simulink library "CTRL_TRGT_YRUPPB"  (R2023b)
settings: Solver=VariableStepAuto  StartTime=0.0  StopTime=10.0  RelTol=1e-3
undefined symbols (not defined in the file or in its folder): c_GravConst_mps2, CTRL_TRGT_YRUPPB_p_Fct1_na
libraries: VUT_lib x1
settings Model: Creator=blatak  LastModifiedBy=blatak

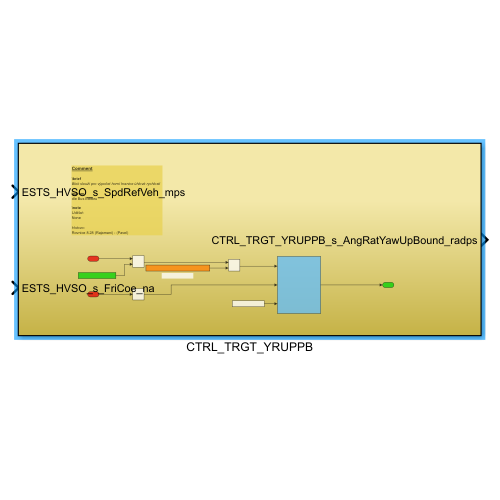
[thumbnail: Simulink's stored preview of the top-level diagram]
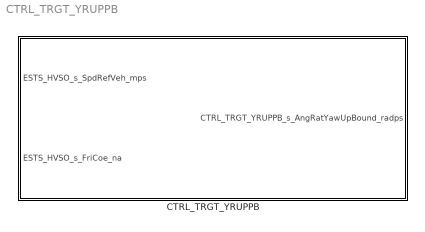
== system CTRL_TRGT_YRUPPB ==
  CTRL_TRGT_YRUPPB : Subsystem

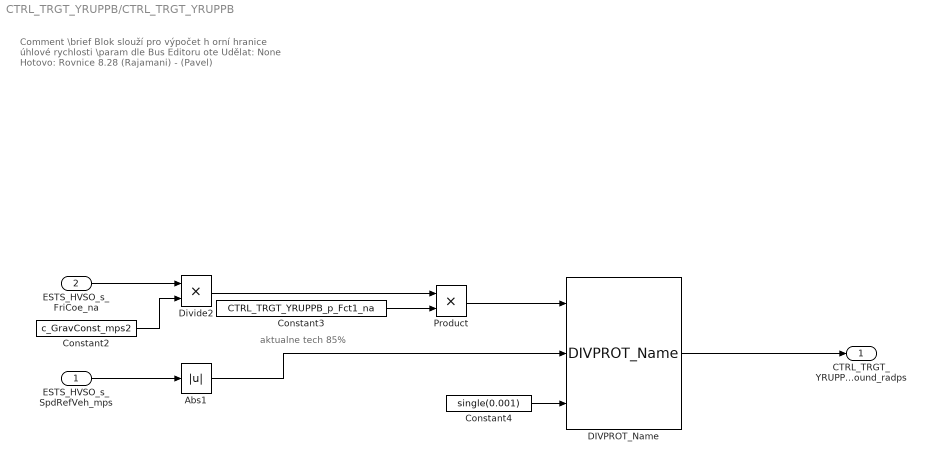
== system CTRL_TRGT_YRUPPB/CTRL_TRGT_YRUPPB ==
  note: aktualne tech 85%
  note: Comment
      |
      | \brief
      | Blok slouží pro výpočet h orní hranice úhlové rychlosti
      |
      | \param
      | dle Bus Editoru
      |
      | \note
      | Udělat:
      | None
      |
      | Hotovo:
      | Rovnice 8.28 (Rajamani) - (Pavel)
  ESTS_HVSO_s_SpdRefVeh_mps : Inport
  ESTS_HVSO_s_FriCoe_na : Inport  Port=2
  Abs1 : Abs  SaturateOnIntegerOverflow=off
  Constant2 : Constant  Value=c_GravConst_mps2
  Constant3 : Constant  Value=CTRL_TRGT_YRUPPB_p_Fct1_na
  Constant4 : Constant  Value=single(0.001)
  DIVPROT_Name : VUT_lib/DIVPROT_Name  SystemSampleTime=-1  VariantActivationTime=update diagram  AllowFlexibleInterface=on  Latency=0  AutoFrameSizeCalculation=off
  Divide2 : Product  Inputs=**
  Product : Product
  CTRL_TRGT_YRUPPB_s_AngRatYawUpBound_radps : Outport
  wires:
  ESTS_HVSO_s_SpdRefVeh_mps/1 -> Abs1/1
  ESTS_HVSO_s_FriCoe_na/1 -> Divide2/1
  Constant2/1 -> Divide2/2
  Divide2/1 -> Product/1
  Constant3/1 -> Product/2
  Product/1 -> DIVPROT_Name/1
  Abs1/1 -> DIVPROT_Name/2
  Constant4/1 -> DIVPROT_Name/3
  DIVPROT_Name/1 -> CTRL_TRGT_YRUPPB_s_AngRatYawUpBound_radps/1
